simulink model "qbot_joystick_nav"  (R2022b)
settings: Solver=ode1  StartTime=0.0  StopTime=inf  FixedStep=1/30  RelTol=1e-3  EnableMultiTasking=on
undefined symbols (not defined in the file): gcbh, Host, JPEG, Point, qc_get_step_size, Video3D, video_display_show
libraries: quarc_library x30
settings Model: SimulationMode=external  ExtModeTrigDuration=10000  Creator=mbohra  LastModifiedBy=mbohra
settings SolverCC: AlgebraicLoopSolver=TrustRegion  PositivePriorityOrder=on
settings DataIOCC: ReturnWorkspaceOutputs=off
settings DebuggingCC: UnconnectedInputMsg=warning  UnconnectedOutputMsg=warning  UnconnectedLineMsg=warning  SFMachineParentedDataDiag=warning  ArithmeticOperatorsInVariantConditions=warning
settings HardwareCC: ProdBitPerLong=64  ProdLargestAtomicInteger=LongLong  ProdLargestAtomicFloat=Double  ProdLongLongMode=on  ProdHWDeviceType=ARM Compatible->ARM 64-bit (LP64)
settings ModelReferenceCC: EnableRefExpFcnMdlSchedulingChecks=on
settings SFSimCC: SimUseLocalCustomCode=off  CustomCodeUndefinedFunction=UseInterfaceOnly
settings RTWCC: Description=QUARC Linux Raspberry Pi Arm64 Target (QBot Platform) Using Toolchain  SystemTargetFile=quarc_linux_pi_arm64.tlc  TemplateMakefile=quarc_default_tmf  RTWUseLocalCustomCode=off  Toolchain=QUARC linux_pi_arm64 | gmake (64-bit Windows)  BuildConfiguration=Faster Runs
settings CodeAppCC: StateflowObjectComments=on
settings STFCustomTargetCC: TargetLangStandard=C99 (ISO)  ConcurrentExecutionCompliant=on  GRTInterface=on  UseToolchainInfoCompliant=on  SystemTargetFile=quarc_linux_pi_arm64.tlc
settings GRTTargetCC: ParMdlRefBuildCompliant=off  CompOptLevelCompliant=off  CombineOutputUpdateFcns=off  MatFileLogging=off  CPPClassGenCompliant=off  GRTInterface=on  ExtMode=on  ExtModeMexFile=quarc_comm  ExtModeMexArgs='-w -d /tmp -uri %u','tcpip://192.168.2.10:17002'
settings ConfigComp: CovMetricSettings=dswe

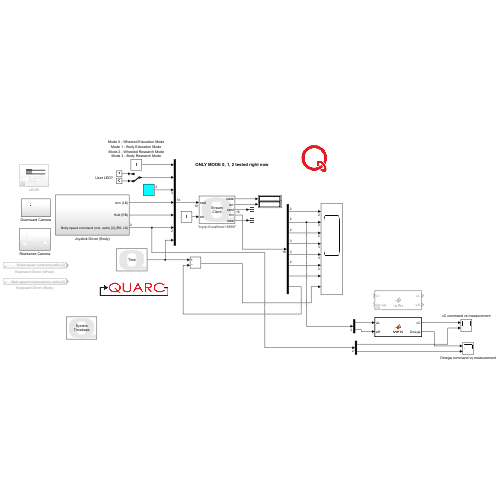
[thumbnail: Simulink's stored preview of the top-level diagram]
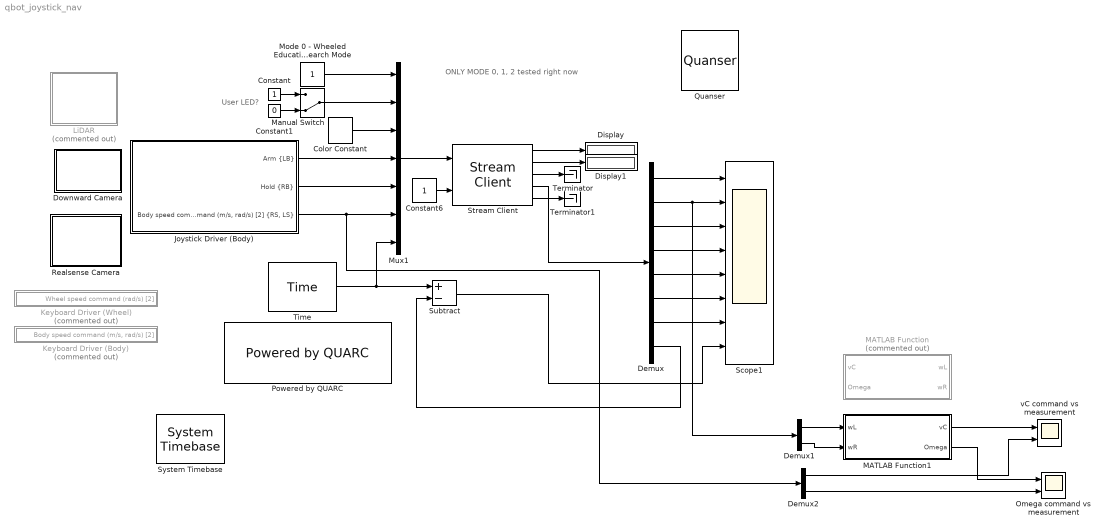
== system qbot_joystick_nav ==
  note: ONLY MODE 0, 1, 2 tested right now
  note: User LED?
  Color Constant : quarc_library/Sources/Signals/Color Constant  color=[0 1 1]
      settings: SourceProductName=QUARC Targets
  Constant : Constant
  Constant1 : Constant  Value=0
  Constant6 : Constant
  Demux : Demux  Outputs=[2 2 2 3 3 2 1 1]
  Demux1 : Demux  Outputs=2
  Demux2 : Demux  Outputs=2
  Display : Display
  Display1 : Display
  Downward Camera : Subsystem
  Joystick Driver (Body) : Subsystem
  Keyboard Driver (Body) : Subsystem  Commented=on
  Keyboard Driver (Wheel) : Subsystem  Commented=on
  LiDAR : Subsystem  Commented=on
  MATLAB Function : MATLAB Function  Commented=on  TreatAsAtomicUnit=on
  MATLAB Function1 : MATLAB Function  TreatAsAtomicUnit=on
  Manual Switch : ManualSwitch  CurrentSetting=0
  Mode 0 - Wheeled Education Mode Mode 1 - Body Education Mode Mode 2 - Wheeled Research Mode Mode 3 - Body Research Mode : Constant
  Mux1 : Mux  Inputs=7
  Omega command vs measurement : Scope  NumInputPorts=2
  Powered by QUARC : quarc_library/Logos/Powered by QUARC
  Quanser : quarc_library/Logos/Quanser
  Realsense Camera : Subsystem
  Scope1 : Scope  NumInputPorts=8
  Stream Client : quarc_library/Communications/Basic/Stream Client  uri_source=Specify via dialog (do not evaluate)  uri=tcpip://localhost:18888  send_buffer_size=1460  receive_buffer_size=1460  byte_order=little endian (Intel - LSB first)  optimization=Minimum latency  send_options=Send most recent data  receive_options=Receive most recent data  default_value=zeros(16,1)  sample_time=qc_get_step_size  active=on  implementation=Use blocking I/O in a separate thread  send_fifo_size=1000  receive_fifo_size=1000  send_priority=0  receive_priority=0  send_dimensions=off  receive_dimensions=off  max_dimensions=-1  data_type=Inherited via back propagation  type_expr=BusObject
      settings: AttributesFormatString="\"tcpip://localhost:18888\""
  Subtract : Sum  Inputs=+-
  System Timebase : quarc_library/Advanced/Timing/System Timebase  stop_on_overrun=off
      settings: SourceProductName=QUARC Targets
  Terminator : Terminator
  Terminator1 : Terminator
  Time : quarc_library/Sources/Time/Time  time_source=Wall clock  sample_time=qc_get_step_size
  vC command vs measurement : Scope  NumInputPorts=2
  wires:
  Mode 0 - Wheeled Education Mode Mode 1 - Body Education Mode Mode 2 - Wheeled Research Mode Mode 3 - Body Research Mode/1 -> Mux1/1
  Manual Switch/1 -> Mux1/2
  Constant/1 -> Manual Switch/1
  Constant1/1 -> Manual Switch/2
  Color Constant/1 -> Mux1/3
  Mux1/1 -> Stream Client/1
  Constant6/1 -> Stream Client/2
  Stream Client/1 -> Display/1
  Stream Client/2 -> Display1/1
  Stream Client/4 -> Demux/1
  Demux/1 -> Scope1/1
  Demux/2 -> Demux1/1, Scope1/2
  Demux/3 -> Scope1/3
  Demux/4 -> Scope1/4
  Demux/5 -> Scope1/5
  Demux/7 -> Scope1/7
  Stream Client/3 -> Terminator/1
  Stream Client/5 -> Terminator1/1
  Time/1 -> Mux1/7, Subtract/1
  Demux/8 -> Subtract/2
  Subtract/1 -> Scope1/8
  Joystick Driver (Body)/2("Hold {RB}") -> Mux1/5
  Joystick Driver (Body)/1("Arm {LB}") -> Mux1/4
  Joystick Driver (Body)/3("Body speed command (m/s, rad/s) [2] {RS, LS}") -> Demux2/1, Mux1/6
  Demux/6 -> Scope1/6
  Demux1/1 -> MATLAB Function1/1(wL)
  Demux1/2 -> MATLAB Function1/2(wR)
  MATLAB Function1/2(Omega) -> Omega command vs measurement/1
  Demux2/2 -> Omega command vs measurement/2
  MATLAB Function1/1(vC) -> vC command vs measurement/1
  Demux2/1 -> vC command vs measurement/2

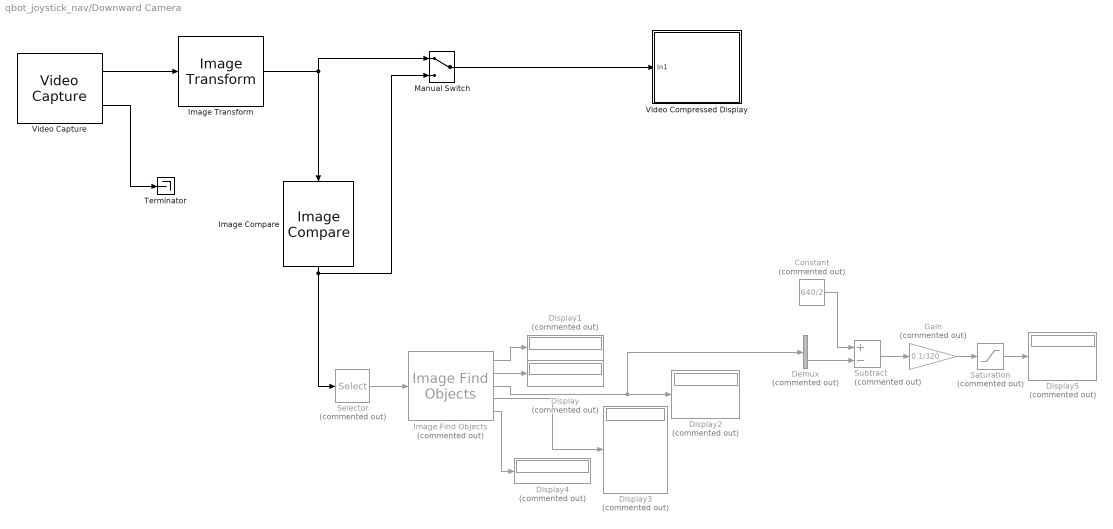
== system qbot_joystick_nav/Downward Camera ==
  Constant : Constant  Commented=on  Value=640/2
  Demux : Demux  Commented=on  Outputs=2
  Display{,1..5} (6 alike) : Display  Commented=on
  Gain : Gain  Commented=on  Gain=0.1/320
  Image Compare : quarc_library/Image Processing/Generic/Image Compare  output_type=Per plane color image (one HxWx3 output)  source=Internal dialog parameters  r_comparison=min <= pixel and pixel <= max  r_minimum=220  r_maximum=255  g_comparison=min <= pixel and pixel <= max  g_minimum=0  g_maximum=64  b_comparison=min <= pixel and pixel <= max  b_minimum=0  b_maximum=200
      settings: SourceProductName=QUARC Targets
  Image Find Objects : quarc_library/Image Processing/Generic/Image Find Objects  Commented=on  num_objects=1  connectivity=8 directions (N, NE, E, SE, S, SW, W, NW)  sort_order=Sort by number of pixels  min_pixels=4000  max_pixels=intmax('uint32')  largest=on  exclude_at_edges=off  variable_size=off  use_complex=off
      settings: SourceProductName=QUARC Targets
  Image Transform : quarc_library/Image Processing/Generic/Image Transform  algorithm=Lens undistort  color_theme=KRYGCBMW  min_pixel=0  max_pixel=4000  focal_length=[302.1629, 301.7493]  principal_point=[185.6271, 306.7551]  radial_coeffs=[-0.3138 0.0780]  tangential_coeffs=[]  extrapolated_pixel=0  interpolation=nearest  row_coords=0  column_coords=0  output_height=480  output_width=640  angle=0  origin=[240 320]  output_origin=[240 320]  output_data_type=uint8
      settings: AttributesFormatString=(%<algorithm>)  SourceProductName=QUARC Targets
  Manual Switch : ManualSwitch
  Saturation : Saturate  Commented=on
  Selector : Selector  Commented=on  NumberOfDimensions=2  InputPortWidth=3  IndexOptions=Index vector (dialog),Select all  Indices=[1:100],1  OutputSizes=1,1
  Subtract : Sum  Commented=on  Inputs=+-
  Terminator : Terminator
  Video Capture : quarc_library/Multimedia/Video Capture  source=device  device=6@tcpip://localhost:18915  filename=sample_movie.mov  value=[0 0; 0 0]  resolution=640 x 480  width=640  height=480  output_format=MATLAB greyscale (HxW)  data_type=uint8  sample_time=qc_get_step_size  brightness_override=off  brightness=50.0  contrast_override=off  contrast=50.0  hue_override=off  hue=50.0  saturation_override=off  saturation=50.0  sharpness_override=off  sharpness=50.0  gamma_override=off  gamma=50.0  coloreffect_override=off  coloreffect=None  whitebalance_override=off  whitebalance=50.0  backlightcompensation_override=off  backlightcompensation=0.0  gain_override=on  gain=98.0  pan_override=off  pan=50.0  tilt_override=off  tilt=50.0  roll_override=off  roll=50.0  zoom_override=off  zoom=0.0  exposure_override=off  exposure=50.0  iris_override=off  iris=50.0  mirror_override=off  mirror=None  focus_override=off  focus=0.0
      settings: SourceProductName=QUARC Targets
  Video Compressed Display : Subsystem  LoadFcn=set_param(gcbh, 'UserData', gcb);  StartFcn=video_display_show([gcb, '/Video Display'], 'add', gcb);  mask(Video Compressed Display){algorithm=JPEG, quality=50, sample_time=-1, use_hardware=on}
      mask prompts: algorithm "Compression algorithm:"; quality "Compression quality (0-100):"; sample_time "Sample time (seconds):"; use_hardware "Use hardware acceleration for video display"
      mask help: Displays a video stream on the host, using compression to minimize bandwidth.
      mask init:
      | qc_set_display('Video\nCompressed\nDisplay');
      settings: UndoDeleteFcn=set_param(gcbh, 'UserData', gcb);  OpenFcn=video_display_show([gcb, '/Video Display'], 'show', gcb);  PreDeleteFcn=video_display_show([gcb, '/Video Display'], 'delete');
      settings: CopyFcn=|
      | set_param(gcbh, 'UserData', gcb);
      | set_param(gcbh, 'LinkStatus', 'none');
      settings: NameChangeFcn=|
      | video_display_show([get_param(gcbh, 'UserData'), '/Video Display'], 'rename', [gcb, '/Video Display']);
      | video_display_show([gcb, '/Video Display'], 'add', gcb);
      | set_param(gcbh, 'UserData', gcb);
      mask Help: web(qc_get_block_help_path(gcb));
      mask TypeOptions algorithm: Image Compress/algorithm
      mask TypeOptions quality: Image Compress/quality
      mask TypeOptions sample_time: Video Display/sample_time
      mask TypeOptions use_hardware: Video Display/use_hardware
      mask Display:
      | patch([0.98591 0.98591 0.62618 0.59072 0.56147   0.536   0.536  0.5441 0.56912 0.59207 0.60881 0.62276 0.63527 0.64364  0.6485  0.6485 0.64706 0.64499 0.63662 0.62411 0.61232 0.59837 0.58307 0.56147   0.536   0.536  0.5441  0.5747 0.60953 0.63662 0.67001  0.7034 0.72851 0.75425 0.77927 0.80294 0.82454 0.84119 0.85865 0.87395 0.88574 0.89339  0.8969 0.89969 0.89969 0.89267  0.8816 0.87044 0.85649  0.8384 0.81824 0.80294 0.78764 0.77513 0.76676 0.75776 0.76397 0.77513 0.79178 0.80987 0.82796 0.84326 0.86207 0.98528],[0.18689 0.05522 0.05522 0.05171 0.05171    0.05 0.18338 0.18338 0.19148 0.20435 0.22298 0.24863 0.28589 0.33125 0.38138 0.55139 0.59801 0.63761 0.68189 0.72149 0.74939 0.76694 0.77855 0.79367 0.79952 0.92768 0.92768 0.92768 0.92417 0.92066 0.91364  0.9032 0.89384 0.88106 0.86594 0.85073 0.82634 0.80537 0.77855 0.74363 0.70403 0.65858 0.61079 0.59099 0.41513 0.37202 0.31847 0.29048 0.25556 0.23342  0.2102 0.19382 0.18221 0.17285 0.16943 0.16124  0.1589 0.16241 0.16709 0.17168  0.1787 0.18221 0.18689 0.18689],[0.9,0.90,0.91])
      | patch([0.536 0.52601 0.46823 0.44528 0.41603 0.39101 0.35555 0.33116 0.31451 0.29291  0.2804 0.26717 0.25322 0.23999 0.22406 0.20732 0.19337 0.17528 0.15935 0.14396 0.13217 0.11759 0.10922 0.10085 0.09671 0.09392 0.09041 0.08906 0.08906 0.09464  0.0995 0.10778 0.11894 0.13145 0.14675 0.16349 0.17672 0.19409 0.20732 0.22406 0.23999 0.26159 0.27833 0.29849 0.31793 0.33602 0.35411 0.37085 0.39245 0.41603   0.536   0.536 0.53159 0.46409   0.446 0.42026 0.39587 0.37571 0.36113 0.34925 0.34088 0.33809 0.33809 0.34088 0.34583 0.35627 0.36392 0.38129 0.39587 0.41117 0.42719 0.44672  0.4676 0.48353 0.48353 0.52394   0.536],[0.05 0.04829 0.04712 0.04712 0.04829 0.05063 0.05405 0.05873 0.06107 0.06692 0.07043 0.07619 0.08087 0.08672 0.09482 0.10652 0.11696 0.13325  0.1508 0.17168 0.19499 0.22415 0.25439 0.28472 0.31379 0.35456 0.38489 0.41513 0.58055 0.63878 0.68774 0.72149 0.75641 0.78089 0.80537 0.82859 0.84029 0.85658 0.86594 0.87404  0.8834 0.89267 0.90086 0.90788 0.91247 0.91832 0.92066   0.923 0.92651 0.92768 0.92768 0.79952 0.79952 0.79952 0.79718 0.78899 0.77153 0.75056 0.72149 0.68072 0.62249  0.5549 0.41396 0.37085 0.33242 0.28121 0.25205 0.22181 0.20552 0.19499 0.18572 0.18221 0.17753 0.17636 0.17753  0.1787  0.1787],[0.9,0.90,0.91])
      | disp('Video\nCompressed\nDisplay');
  wires:
  Video Capture/2 -> Terminator/1
  Video Capture/1 -> Image Transform/1
  Image Transform/1 -> Manual Switch/1, Image Compare/1
  Selector/1 -> Image Find Objects/1
  Image Find Objects/2 -> Display/1
  Image Find Objects/1 -> Display1/1
  Image Find Objects/3 -> Demux/1, Display2/1
  Image Find Objects/4 -> Display3/1
  Image Find Objects/5 -> Display4/1
  Image Compare/1 -> Selector/1, Manual Switch/2
  Manual Switch/1 -> Video Compressed Display/1(In1)
  Demux/2 -> Subtract/2
  Constant/1 -> Subtract/1
  Saturation/1 -> Display5/1
  Subtract/1 -> Gain/1
  Gain/1 -> Saturation/1

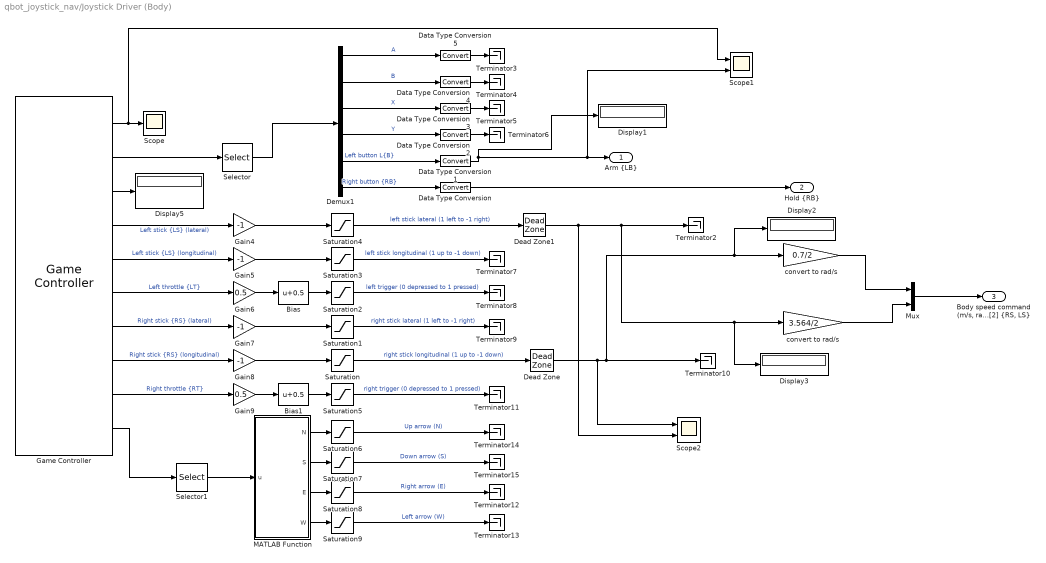
== system qbot_joystick_nav/Joystick Driver (Body) ==
  Bias : Bias  Bias=0.5  SaturateOnIntegerOverflow=off
  Bias1 : Bias  Bias=0.5  SaturateOnIntegerOverflow=off
  Data Type Conversion{,1..5} (6 alike) : DataTypeConversion  SaturateOnIntegerOverflow=off  RndMeth=Floor
  Dead Zone : DeadZone  LowerValue=-0.05  UpperValue=0.05
  Dead Zone1 : DeadZone  LowerValue=-0.05  UpperValue=0.05
  Demux1 : Demux  Outputs=6
  Display{1..3,5} (4 alike) : Display
  Gain{4..5,7..8} (4 alike) : Gain  Gain=-1
  Gain6 : Gain  Gain=0.5
  Gain9 : Gain  Gain=0.5
  Game Controller : quarc_library/Devices/Peripherals/Target/Game Controller  controller=1  buffer_size=12  deadzone=[]  saturation=[]  sample_time=qc_get_step_size  auto_center=off  enabled=on
      settings: SourceProductName=QUARC Targets
  MATLAB Function : MATLAB Function  TreatAsAtomicUnit=on
  Mux : Mux  Inputs=2
  Saturation{,1,3..4} (4 alike) : Saturate  UpperLimit=1  LowerLimit=-1
  Saturation{2,5..9} (6 alike) : Saturate  UpperLimit=1  LowerLimit=0
  Scope : Scope
  Scope1 : Scope  NumInputPorts=2
  Scope2 : Scope  NumInputPorts=2
  Selector : Selector  InputPortWidth=32  IndexOptions=Index vector (dialog)  Indices=[1:6]  OutputSizes=1
  Selector1 : Selector  InputPortWidth=4  IndexOptions=Index vector (dialog)  Indices=1  OutputSizes=1
  Terminator{2..15} (14 alike) : Terminator
  convert to rad/s : Gain  Gain=0.7/2
  "convert to rad/s " : Gain  Gain=3.564/2
  "Arm {LB}" : Outport
  "Hold {RB}" : Outport  Port=2
  "Body speed command (m/s, rad/s) [2] {RS, LS}" : Outport  Port=3
  wires:
  convert to rad/s/1 -> Mux/1
  Mux/1 -> "Body speed command (m/s, rad/s) [2] {RS, LS}"/1
  Game Controller/1 -> Scope1/1, Scope/1
  Game Controller/2 -> Selector/1
  Game Controller/3 -> Display5/1
  Game Controller/4 -> Gain4/1  "Left stick {LS} (lateral)"
  Game Controller/5 -> Gain5/1  "Left stick {LS} (longitudinal)"
  Game Controller/6 -> Gain6/1  "Left throttle {LT}"
  Game Controller/7 -> Gain7/1  "Right stick {RS} (lateral)"
  Game Controller/8 -> Gain8/1  "Right stick {RS} (longitudinal)"
  Game Controller/9 -> Gain9/1  "Right throttle {RT}"
  Game Controller/10 -> Selector1/1
  Selector/1 -> Demux1/1
  Demux1/1 -> Data Type Conversion5/1  "A"
  Demux1/2 -> Data Type Conversion4/1  "B"
  Demux1/3 -> Data Type Conversion3/1  "X"
  Demux1/4 -> Data Type Conversion2/1  "Y"
  Demux1/5 -> Data Type Conversion1/1  "Left button L{B}"
  Demux1/6 -> Data Type Conversion/1  "Right button {RB}"
  Selector1/1 -> MATLAB Function/1(u)
  Gain6/1 -> Bias/1
  Gain9/1 -> Bias1/1
  Gain8/1 -> Saturation/1
  Gain7/1 -> Saturation1/1
  Gain5/1 -> Saturation3/1
  Gain4/1 -> Saturation4/1
  Bias/1 -> Saturation2/1
  Bias1/1 -> Saturation5/1
  Saturation4/1 -> Dead Zone1/1  "left stick lateral (1 left to -1 right)"
  Saturation3/1 -> Terminator7/1  "left stick longitudinal (1 up to -1 down)"
  Saturation2/1 -> Terminator8/1  "left trigger (0 depressed to 1 pressed)"
  Saturation1/1 -> Terminator9/1  "right stick lateral (1 left to -1 right)"
  Saturation/1 -> Dead Zone/1  "right stick longitudinal (1 up to -1 down)"
  Saturation5/1 -> Terminator11/1  "right trigger (0 depressed to 1 pressed)"
  MATLAB Function/1(N) -> Saturation6/1
  MATLAB Function/2(S) -> Saturation7/1
  MATLAB Function/3(E) -> Saturation8/1
  MATLAB Function/4(W) -> Saturation9/1
  Saturation6/1 -> Terminator14/1  "Up arrow (N)"
  Saturation7/1 -> Terminator15/1  "Down arrow (S)"
  Saturation8/1 -> Terminator12/1  "Right arrow (E)"
  Saturation9/1 -> Terminator13/1  "Left arrow (W)"
  Data Type Conversion1/1 -> Display1/1, Scope1/2, "Arm {LB}"/1
  Data Type Conversion2/1 -> Terminator6/1
  Data Type Conversion3/1 -> Terminator5/1
  Data Type Conversion4/1 -> Terminator4/1
  Data Type Conversion5/1 -> Terminator3/1
  Data Type Conversion/1 -> "Hold {RB}"/1
  "convert to rad/s "/1 -> Mux/2
  Dead Zone/1 -> Scope2/1, convert to rad/s/1, Display2/1, Terminator10/1
  Dead Zone1/1 -> Scope2/2, "convert to rad/s "/1, Display3/1, Terminator2/1

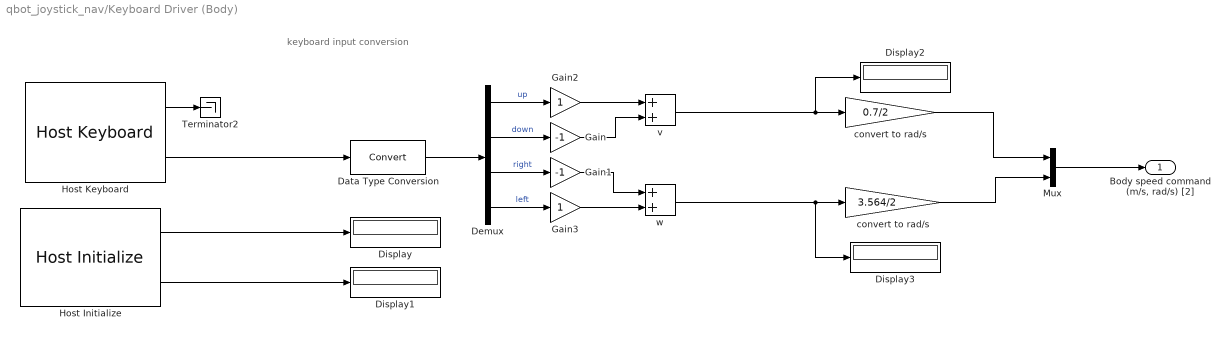
== system qbot_joystick_nav/Keyboard Driver (Body) ==
  note: keyboard input conversion
  Data Type Conversion : DataTypeConversion  SaturateOnIntegerOverflow=off  RndMeth=Floor
  Demux : Demux
  Display{,1..3} (4 alike) : Display
  Gain : Gain  Gain=-1
  Gain1 : Gain  Gain=-1
  Gain2 : Gain
  Gain3 : Gain
  Host Initialize : quarc_library/Devices/Peripherals/Host/Host Initialize  object_name=Host-2  uri_source=Use external mode communications  uri=tcpip://localhost:18001  send_buffer_size=1000  receive_buffer_size=1000  thread_priority=0  run_client=on  use_window=off  window_position=[]  sample_time=qc_get_step_size  active=on
      settings: SourceProductName=QUARC Targets
  Host Keyboard : quarc_library/Devices/Peripherals/Host/Host Keyboard  object_name=Host-2  virtual_key="[38  40  39  37]"  sample_time=qc_get_step_size  enabled=on  debug_mode=off
      settings: SourceProductName=QUARC Targets
  Mux : Mux  Inputs=2
  Terminator2 : Terminator
  convert to rad/s : Gain  Gain=0.7/2
  "convert to rad/s " : Gain  Gain=3.564/2
  v : Sum
  w : Sum
  "Body speed command (m/s, rad/s) [2]" : Outport
  wires:
  Host Initialize/2 -> Display1/1
  w/1 -> "convert to rad/s "/1, Display3/1
  Host Initialize/1 -> Display/1
  Host Keyboard/1 -> Terminator2/1
  v/1 -> convert to rad/s/1, Display2/1
  Data Type Conversion/1 -> Demux/1
  Gain3/1 -> w/2
  Gain2/1 -> v/1
  Demux/3 -> Gain1/1  "right"
  Demux/4 -> Gain3/1  "left"
  Host Keyboard/2 -> Data Type Conversion/1
  Demux/1 -> Gain2/1  "up"
  Gain/1 -> v/2
  Gain1/1 -> w/1
  Demux/2 -> Gain/1  "down"
  "convert to rad/s "/1 -> Mux/2
  convert to rad/s/1 -> Mux/1
  Mux/1 -> "Body speed command (m/s, rad/s) [2]"/1

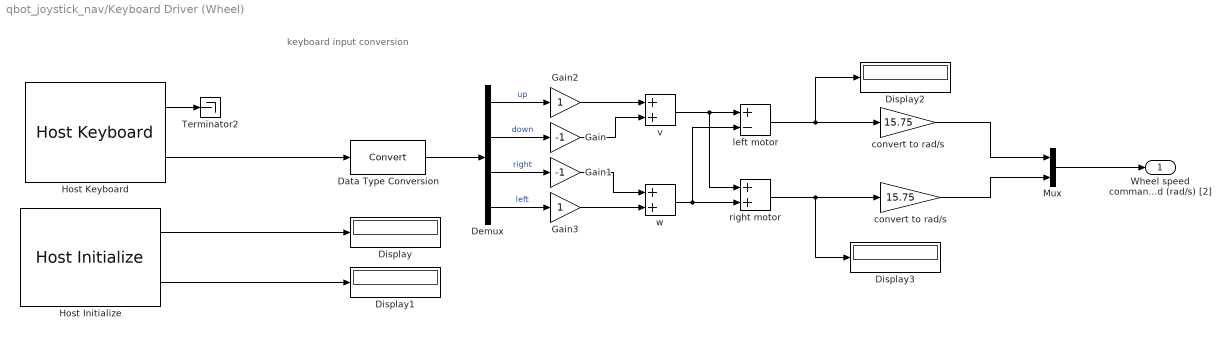
== system qbot_joystick_nav/Keyboard Driver (Wheel) ==
  note: keyboard input conversion
  Data Type Conversion : DataTypeConversion  SaturateOnIntegerOverflow=off  RndMeth=Floor
  Demux : Demux
  Display{,1..3} (4 alike) : Display
  Gain : Gain  Gain=-1
  Gain1 : Gain  Gain=-1
  Gain2 : Gain
  Gain3 : Gain
  Host Initialize : quarc_library/Devices/Peripherals/Host/Host Initialize  object_name=Host-1  uri_source=Use external mode communications  uri=tcpip://localhost:18001  send_buffer_size=1000  receive_buffer_size=1000  thread_priority=0  run_client=on  use_window=off  window_position=[]  sample_time=qc_get_step_size  active=on
      settings: SourceProductName=QUARC Targets
  Host Keyboard : quarc_library/Devices/Peripherals/Host/Host Keyboard  object_name=Host-1  virtual_key="[38  40  39  37]"  sample_time=qc_get_step_size  enabled=on  debug_mode=off
      settings: SourceProductName=QUARC Targets
  Mux : Mux  Inputs=2
  Terminator2 : Terminator
  convert to rad/s : Gain  Gain=15.75
  "convert to rad/s " : Gain  Gain=15.75
  left motor : Sum  Inputs=+-
  right motor : Sum
  v : Sum
  w : Sum
  Wheel speed command (rad/s) [2] : Outport
  wires:
  Host Initialize/2 -> Display1/1
  right motor/1 -> Display3/1, "convert to rad/s "/1
  Host Initialize/1 -> Display/1
  Host Keyboard/1 -> Terminator2/1
  left motor/1 -> convert to rad/s/1, Display2/1
  Data Type Conversion/1 -> Demux/1
  Gain3/1 -> w/2
  Gain2/1 -> v/1
  Demux/3 -> Gain1/1  "right"
  Demux/4 -> Gain3/1  "left"
  Host Keyboard/2 -> Data Type Conversion/1
  v/1 -> right motor/1, left motor/1
  Demux/1 -> Gain2/1  "up"
  w/1 -> left motor/2, right motor/2
  Gain/1 -> v/2
  Gain1/1 -> w/1
  Demux/2 -> Gain/1  "down"
  "convert to rad/s "/1 -> Mux/2
  convert to rad/s/1 -> Mux/1
  Mux/1 -> Wheel speed command (rad/s) [2]/1

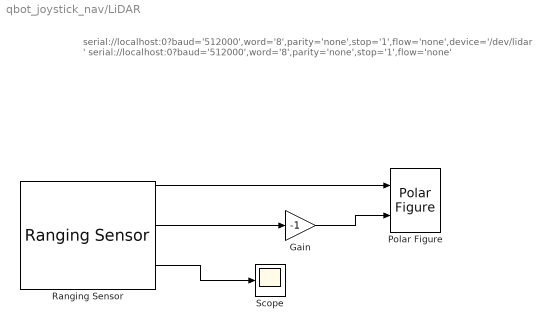
== system qbot_joystick_nav/LiDAR ==
  note: serial://localhost:0?baud='512000',word='8',parity='none',stop='1',flow='none',device='/dev/lidar '
      |
      | serial://localhost:0?baud='512000',word='8',parity='none',stop='1',flow='none'
  Gain : Gain  Gain=-1
  Polar Figure : quarc_library/Sinks/Figures/Polar Figure  figure_mode=Use figure window  figure_tag=figure1  axes_tag=axes1  plot_mode=Frame-based  minimum_rho=0  maximum_rho=8  minimum_theta=0  maximum_theta=360  zero_location=right  direction=counterclockwise  buffer_size=1000  update_rate=1  sample_time=-1  initial_position="2  566  958  457"  initial_visibility=on  line1_style=None  line1_width=0.5  line1_color=[0 0.4470 0.7410]  marker1=Point (.)  marker1_size=6  marker1_edge_color=[0 0.447059 0.741176]  marker1_face_color=[0 0.447059 0.741176]  line2_style=Solid line (-)  line2_width=0.5  line2_color=[0.85098 0.32549 0.0980392]  marker2=None  marker2_size=6  marker2_edge_color=[0.85098 0.32549 0.0980392]  marker2_face_color=[0.85098 0.32549 0.0980392]  line3_style=Solid line (-)  line3_width=0.5  line3_color=[0.929412 0.694118 0.12549]  marker3=None  marker3_size=6  marker3_edge_color=[0.929412 0.694118 0.12549]  marker3_face_color=[0.929412 0.694118 0.12549]  line4_style=Solid line (-)  line4_width=0.5  line4_color=[0.494118 0.184314 0.556863]  marker4=None  marker4_size=6  marker4_edge_color=[0.494118 0.184314 0.556863]  marker4_face_color=[0.494118 0.184314 0.556863]  line5_style=Solid line (-)  line5_width=0.5  line5_color=[0.466667 0.67451 0.188235]  marker5=None  marker5_size=6  marker5_edge_color=[0.466667 0.67451 0.188235]  marker5_face_color=[0.466667 0.67451 0.188235]
      settings: SourceProductName=QUARC Targets
  Ranging Sensor : quarc_library/Devices/Third-Party/Sensors/Ranging Sensor  sensor_type=Leishen M10P LIDAR  uri=serial://localhost:0?baud='512000',word='8',parity='none',stop='1',flow='none',device='/dev/lidar'  ranging_distance=Short  timing_budget=0.033  measurement_period=0.0005  output_mode=Fixed-size output  samples_per_revolution=1680  max_distance=0.050  max_angle=5  sample_time=qc_get_step_size*3  show_versions=off  active=on
      settings: SourceProductName=QUARC Targets
  Scope : Scope
  wires:
  Ranging Sensor/3 -> Gain/1
  Gain/1 -> Polar Figure/2
  Ranging Sensor/1 -> Polar Figure/1
  Ranging Sensor/5 -> Scope/1

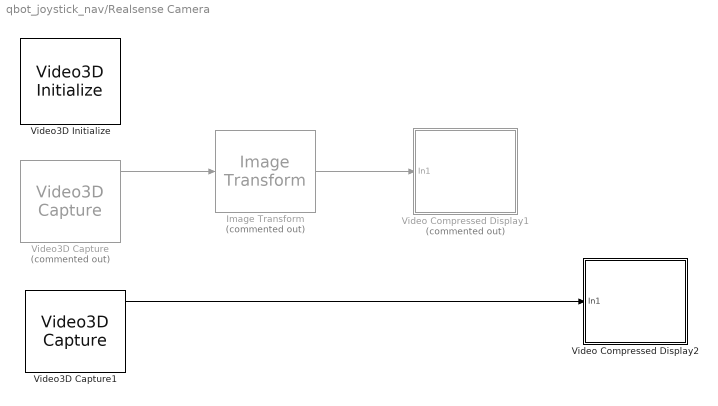
== system qbot_joystick_nav/Realsense Camera ==
  Image Transform : quarc_library/Image Processing/Generic/Image Transform  Commented=on  algorithm=Colorize  color_theme=KRYGCBMW  min_pixel=0  max_pixel=4000  focal_length=308  principal_point=[262 334]  radial_coeffs=[-0.3129 0.0907]  tangential_coeffs=[]  extrapolated_pixel=0  interpolation=nearest  row_coords=0  column_coords=0  output_height=480  output_width=640  angle=0  origin=[240 320]  output_origin=[240 320]  output_data_type=uint8
      settings: AttributesFormatString=(%<algorithm>)  SourceProductName=QUARC Targets
  Video Compressed Display1 : Subsystem  Commented=on  LoadFcn=set_param(gcbh, 'UserData', gcb);  StartFcn=video_display_show([gcb, '/Video Display'], 'add', gcb);  mask(Video Compressed Display){algorithm=JPEG, quality=50, sample_time=-1, use_hardware=on}
      mask prompts: algorithm "Compression algorithm:"; quality "Compression quality (0-100):"; sample_time "Sample time (seconds):"; use_hardware "Use hardware acceleration for video display"
      mask help: Displays a video stream on the host, using compression to minimize bandwidth.
      mask init:
      | qc_set_display('Video\nCompressed\nDisplay');
      settings: UndoDeleteFcn=set_param(gcbh, 'UserData', gcb);  OpenFcn=video_display_show([gcb, '/Video Display'], 'show', gcb);  PreDeleteFcn=video_display_show([gcb, '/Video Display'], 'delete');
      settings: CopyFcn=|
      | set_param(gcbh, 'UserData', gcb);
      | set_param(gcbh, 'LinkStatus', 'none');
      settings: NameChangeFcn=|
      | video_display_show([get_param(gcbh, 'UserData'), '/Video Display'], 'rename', [gcb, '/Video Display']);
      | video_display_show([gcb, '/Video Display'], 'add', gcb);
      | set_param(gcbh, 'UserData', gcb);
      mask Help: web(qc_get_block_help_path(gcb));
      mask TypeOptions algorithm: Image Compress/algorithm
      mask TypeOptions quality: Image Compress/quality
      mask TypeOptions sample_time: Video Display/sample_time
      mask TypeOptions use_hardware: Video Display/use_hardware
      mask Display:
      | patch([0.98591 0.98591 0.62618 0.59072 0.56147   0.536   0.536  0.5441 0.56912 0.59207 0.60881 0.62276 0.63527 0.64364  0.6485  0.6485 0.64706 0.64499 0.63662 0.62411 0.61232 0.59837 0.58307 0.56147   0.536   0.536  0.5441  0.5747 0.60953 0.63662 0.67001  0.7034 0.72851 0.75425 0.77927 0.80294 0.82454 0.84119 0.85865 0.87395 0.88574 0.89339  0.8969 0.89969 0.89969 0.89267  0.8816 0.87044 0.85649  0.8384 0.81824 0.80294 0.78764 0.77513 0.76676 0.75776 0.76397 0.77513 0.79178 0.80987 0.82796 0.84326 0.86207 0.98528],[0.18689 0.05522 0.05522 0.05171 0.05171    0.05 0.18338 0.18338 0.19148 0.20435 0.22298 0.24863 0.28589 0.33125 0.38138 0.55139 0.59801 0.63761 0.68189 0.72149 0.74939 0.76694 0.77855 0.79367 0.79952 0.92768 0.92768 0.92768 0.92417 0.92066 0.91364  0.9032 0.89384 0.88106 0.86594 0.85073 0.82634 0.80537 0.77855 0.74363 0.70403 0.65858 0.61079 0.59099 0.41513 0.37202 0.31847 0.29048 0.25556 0.23342  0.2102 0.19382 0.18221 0.17285 0.16943 0.16124  0.1589 0.16241 0.16709 0.17168  0.1787 0.18221 0.18689 0.18689],[0.9,0.90,0.91])
      | patch([0.536 0.52601 0.46823 0.44528 0.41603 0.39101 0.35555 0.33116 0.31451 0.29291  0.2804 0.26717 0.25322 0.23999 0.22406 0.20732 0.19337 0.17528 0.15935 0.14396 0.13217 0.11759 0.10922 0.10085 0.09671 0.09392 0.09041 0.08906 0.08906 0.09464  0.0995 0.10778 0.11894 0.13145 0.14675 0.16349 0.17672 0.19409 0.20732 0.22406 0.23999 0.26159 0.27833 0.29849 0.31793 0.33602 0.35411 0.37085 0.39245 0.41603   0.536   0.536 0.53159 0.46409   0.446 0.42026 0.39587 0.37571 0.36113 0.34925 0.34088 0.33809 0.33809 0.34088 0.34583 0.35627 0.36392 0.38129 0.39587 0.41117 0.42719 0.44672  0.4676 0.48353 0.48353 0.52394   0.536],[0.05 0.04829 0.04712 0.04712 0.04829 0.05063 0.05405 0.05873 0.06107 0.06692 0.07043 0.07619 0.08087 0.08672 0.09482 0.10652 0.11696 0.13325  0.1508 0.17168 0.19499 0.22415 0.25439 0.28472 0.31379 0.35456 0.38489 0.41513 0.58055 0.63878 0.68774 0.72149 0.75641 0.78089 0.80537 0.82859 0.84029 0.85658 0.86594 0.87404  0.8834 0.89267 0.90086 0.90788 0.91247 0.91832 0.92066   0.923 0.92651 0.92768 0.92768 0.79952 0.79952 0.79952 0.79718 0.78899 0.77153 0.75056 0.72149 0.68072 0.62249  0.5549 0.41396 0.37085 0.33242 0.28121 0.25205 0.22181 0.20552 0.19499 0.18572 0.18221 0.17753 0.17636 0.17753  0.1787  0.1787],[0.9,0.90,0.91])
      | disp('Video\nCompressed\nDisplay');
  Video Compressed Display2 : Subsystem  LoadFcn=set_param(gcbh, 'UserData', gcb);  StartFcn=video_display_show([gcb, '/Video Display'], 'add', gcb);  mask(Video Compressed Display){algorithm=JPEG, quality=50, sample_time=-1, use_hardware=on}
      mask prompts: algorithm "Compression algorithm:"; quality "Compression quality (0-100):"; sample_time "Sample time (seconds):"; use_hardware "Use hardware acceleration for video display"
      mask help: Displays a video stream on the host, using compression to minimize bandwidth.
      mask init:
      | qc_set_display('Video\nCompressed\nDisplay');
      settings: UndoDeleteFcn=set_param(gcbh, 'UserData', gcb);  OpenFcn=video_display_show([gcb, '/Video Display'], 'show', gcb);  PreDeleteFcn=video_display_show([gcb, '/Video Display'], 'delete');
      settings: CopyFcn=|
      | set_param(gcbh, 'UserData', gcb);
      | set_param(gcbh, 'LinkStatus', 'none');
      settings: NameChangeFcn=|
      | video_display_show([get_param(gcbh, 'UserData'), '/Video Display'], 'rename', [gcb, '/Video Display']);
      | video_display_show([gcb, '/Video Display'], 'add', gcb);
      | set_param(gcbh, 'UserData', gcb);
      mask Help: web(qc_get_block_help_path(gcb));
      mask TypeOptions algorithm: Image Compress/algorithm
      mask TypeOptions quality: Image Compress/quality
      mask TypeOptions sample_time: Video Display/sample_time
      mask TypeOptions use_hardware: Video Display/use_hardware
      mask Display:
      | patch([0.98591 0.98591 0.62618 0.59072 0.56147   0.536   0.536  0.5441 0.56912 0.59207 0.60881 0.62276 0.63527 0.64364  0.6485  0.6485 0.64706 0.64499 0.63662 0.62411 0.61232 0.59837 0.58307 0.56147   0.536   0.536  0.5441  0.5747 0.60953 0.63662 0.67001  0.7034 0.72851 0.75425 0.77927 0.80294 0.82454 0.84119 0.85865 0.87395 0.88574 0.89339  0.8969 0.89969 0.89969 0.89267  0.8816 0.87044 0.85649  0.8384 0.81824 0.80294 0.78764 0.77513 0.76676 0.75776 0.76397 0.77513 0.79178 0.80987 0.82796 0.84326 0.86207 0.98528],[0.18689 0.05522 0.05522 0.05171 0.05171    0.05 0.18338 0.18338 0.19148 0.20435 0.22298 0.24863 0.28589 0.33125 0.38138 0.55139 0.59801 0.63761 0.68189 0.72149 0.74939 0.76694 0.77855 0.79367 0.79952 0.92768 0.92768 0.92768 0.92417 0.92066 0.91364  0.9032 0.89384 0.88106 0.86594 0.85073 0.82634 0.80537 0.77855 0.74363 0.70403 0.65858 0.61079 0.59099 0.41513 0.37202 0.31847 0.29048 0.25556 0.23342  0.2102 0.19382 0.18221 0.17285 0.16943 0.16124  0.1589 0.16241 0.16709 0.17168  0.1787 0.18221 0.18689 0.18689],[0.9,0.90,0.91])
      | patch([0.536 0.52601 0.46823 0.44528 0.41603 0.39101 0.35555 0.33116 0.31451 0.29291  0.2804 0.26717 0.25322 0.23999 0.22406 0.20732 0.19337 0.17528 0.15935 0.14396 0.13217 0.11759 0.10922 0.10085 0.09671 0.09392 0.09041 0.08906 0.08906 0.09464  0.0995 0.10778 0.11894 0.13145 0.14675 0.16349 0.17672 0.19409 0.20732 0.22406 0.23999 0.26159 0.27833 0.29849 0.31793 0.33602 0.35411 0.37085 0.39245 0.41603   0.536   0.536 0.53159 0.46409   0.446 0.42026 0.39587 0.37571 0.36113 0.34925 0.34088 0.33809 0.33809 0.34088 0.34583 0.35627 0.36392 0.38129 0.39587 0.41117 0.42719 0.44672  0.4676 0.48353 0.48353 0.52394   0.536],[0.05 0.04829 0.04712 0.04712 0.04829 0.05063 0.05405 0.05873 0.06107 0.06692 0.07043 0.07619 0.08087 0.08672 0.09482 0.10652 0.11696 0.13325  0.1508 0.17168 0.19499 0.22415 0.25439 0.28472 0.31379 0.35456 0.38489 0.41513 0.58055 0.63878 0.68774 0.72149 0.75641 0.78089 0.80537 0.82859 0.84029 0.85658 0.86594 0.87404  0.8834 0.89267 0.90086 0.90788 0.91247 0.91832 0.92066   0.923 0.92651 0.92768 0.92768 0.79952 0.79952 0.79952 0.79718 0.78899 0.77153 0.75056 0.72149 0.68072 0.62249  0.5549 0.41396 0.37085 0.33242 0.28121 0.25205 0.22181 0.20552 0.19499 0.18572 0.18221 0.17753 0.17636 0.17753  0.1787  0.1787],[0.9,0.90,0.91])
      | disp('Video\nCompressed\nDisplay');
  Video3D Capture : quarc_library/Multimedia/Video3D Capture  Commented=on  object_name=unassigned  stream_type=Depth  stream_index=0  resolution=640 x 480  width=640  height=480  output_format=MATLAB greyscale (HxW)  data_type=uint16  sample_time=qc_get_step_size * 10  camera_intrinsics=off  depth_scale=off  brightness_override=off  brightness=50.0  contrast_override=off  contrast=50.0  hue_override=off  hue=50.0  saturation_override=off  saturation=50.0  sharpness_override=off  sharpness=50.0  gamma_override=off  gamma=50.0  gain_override=off  gain=50.0  backlightcompensation_override=off  backlightcompensation=50.0  whitebalance_override=Automatic white balance  whitebalance=50.0  exposure_override=Automatic exposure  exposure=30.0  emitter=Enable laser emitter  preset=Do not set camera presets
  Video3D Capture1 : quarc_library/Multimedia/Video3D Capture  object_name=Video3D-1  stream_type=RGB  stream_index=0  resolution=640 x 480  width=640  height=480  output_format=MATLAB RGB (HxWx3)  data_type=uint8  sample_time=qc_get_step_size  camera_intrinsics=off  depth_scale=off  brightness_override=off  brightness=50.0  contrast_override=off  contrast=50.0  hue_override=off  hue=50.0  saturation_override=off  saturation=50.0  sharpness_override=off  sharpness=50.0  gamma_override=off  gamma=50.0  gain_override=off  gain=50.0  backlightcompensation_override=off  backlightcompensation=50.0  whitebalance_override=Automatic white balance  whitebalance=50.0  exposure_override=Automatic exposure  exposure=30.0  emitter=Enable laser emitter  preset=Do not set camera presets
  Video3D Initialize : quarc_library/Multimedia/Video3D Initialize  object_name=Video3D-1  source=Device  identifier=0@tcpip://localhost:18917  file=sample.bag  sample_time=qc_get_step_size * ceil(1/30 / qc_get_step_size)  active=on
  wires:
  Video3D Capture1/1 -> Video Compressed Display2/1(In1)
  Video3D Capture/1 -> Image Transform/1
  Image Transform/1 -> Video Compressed Display1/1(In1)

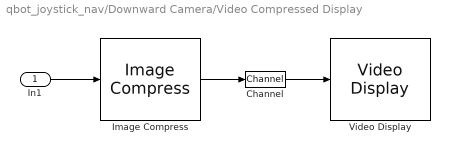
== system qbot_joystick_nav/Downward Camera/Video Compressed Display ==
  In1 : Inport
  Channel : quarc_library/Signal Routing/Channel  channel=0  buffer_size=1
  Image Compress : quarc_library/Image Processing/Generic/Image Compress  algorithm=JPEG  source=Internal dialog parameter  quality=quality  output_dim=-1
  Video Display : quarc_library/Multimedia/Video Display  Tag=qbot_joystick_nav/Downward Camera/Video Compressed Display/Video Display  sample_time=sample_time  use_hardware=on
  wires:
  Image Compress/1 -> Channel/1
  In1/1 -> Image Compress/1
  Channel/1 -> Video Display/1

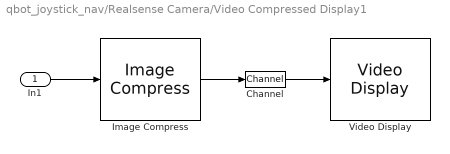
== system qbot_joystick_nav/Realsense Camera/Video Compressed Display1 ==
  In1 : Inport
  Channel : quarc_library/Signal Routing/Channel  channel=0  buffer_size=1
  Image Compress : quarc_library/Image Processing/Generic/Image Compress  algorithm=JPEG  source=Internal dialog parameter  quality=quality  output_dim=-1
  Video Display : quarc_library/Multimedia/Video Display  Tag=qbot_joystick_nav/Realsense Camera/Video Compressed Display1/Video Display  sample_time=sample_time  use_hardware=on
  wires:
  Channel/1 -> Video Display/1
  In1/1 -> Image Compress/1
  Image Compress/1 -> Channel/1

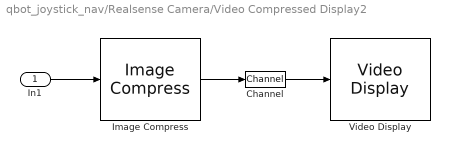
== system qbot_joystick_nav/Realsense Camera/Video Compressed Display2 ==
  In1 : Inport
  Channel : quarc_library/Signal Routing/Channel  channel=1  buffer_size=1
  Image Compress : quarc_library/Image Processing/Generic/Image Compress  algorithm=JPEG  source=Internal dialog parameter  quality=quality  output_dim=-1
  Video Display : quarc_library/Multimedia/Video Display  Tag=qbot_joystick_nav/Realsense Camera/Video Compressed Display2/Video Display  sample_time=sample_time  use_hardware=on
  wires:
  Image Compress/1 -> Channel/1
  In1/1 -> Image Compress/1
  Channel/1 -> Video Display/1

== matlab function qbot_joystick_nav/MATLAB Function ==
  data: vC input; wL output; Omega input; wR output
function [wL, wR] = invKin(vC , Omega)

% wheelbase
d=0.3928; 

% calculate wheel linear velocities
vR = vC + Omega*d/2;
vL = vC - Omega*d/2;

% calculate wheel angular velocities
wheelRadius = 3.5*0.0254/2;

wR = vR/ wheelRadius;
wL = vL/ wheelRadius;

== matlab function qbot_joystick_nav/Joystick Driver (Body)/MATLAB Function ==
  data: u input; N output; S output; E output; W output
function [N, S, E, W] = fcn(u)

N = 0;
S = 0;
E = 0;
W = 0;

switch u
    case 0
        N = 1;
    case 3.142
        S = 1;
    case 4.712
        W = 1;
    case 1.571
        E = 1;
    case 3.927
        S = 1;
        W = 1;
    case 2.356
        S = 1;
        E = 1;
    case 0.7854
        N = 1;
        E = 1;
    case 5.498
        N = 1;
        W = 1;
end

== matlab function qbot_joystick_nav/MATLAB Function1 ==
  data: wL input; vC output; wR input; Omega output
function [vC , Omega] = forKin(wL, wR)

% calculate wheel angular velocities
wheelRadius = 3.5*0.0254/2;

vR = wR * wheelRadius;
vL = wL * wheelRadius;

% wheelbase
d=0.3928; 

% calculate wheel linear velocities
vC = (vR + vL)/2;
Omega = (vR - vL)/d;
